simulink model "BuckDriven_DC_Mot_Offline"  (R2024b)
settings: Solver=VariableStepAuto  StartTime=0.0  StopTime=1  RelTol=1e-3
InitFcn:
  | Vin = 12;
  | 
  | %Buck Parameters
  | L = single(438e-6);
  | C = single(8e-6);
  | RDS = 0.852;
  | RL = single(0.167);
  | RD = single(0.1);
  | ESR = 2.28;
  | VD = 0.75;
  | 
  | overL = 1/L;
  | overC = 1/C;
  | 
  | %Motor Parameters
  | Ra = single(2.461);
  | La = single(0.0351);
  | Rf = single(47.74);
  | Lf = single(0.3364);
  | KLm = single(0.1963);
  | If = single(Vin/Rf);
  | J = single(0.0138);
  | f = single(0.1);
  | Tm = 0;
  | 
  | overLa = 1/La;
  | overJ = 1/J;
  | RaESR = Ra+ESR;
  | K = KLm*If;
  | 
  | vG = 4095/15;
  | wG = 4095/250;
  | 
  | h = 2e-6;
settings Model: Creator=User  LastModifiedBy=User

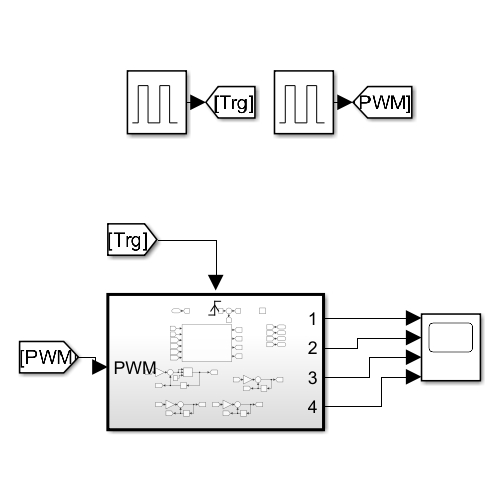
[thumbnail: Simulink's stored preview of the top-level diagram]
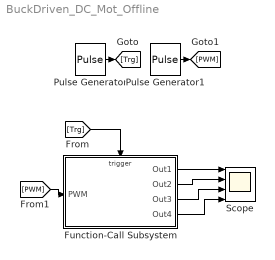
== system BuckDriven_DC_Mot_Offline ==
  Function-Call Subsystem : Subsystem  TreatAsAtomicUnit=on
  Pulse Generator : DiscretePulseGenerator  PulseType=Time based  Period=h  PulseWidth=5
  Pulse Generator1 : DiscretePulseGenerator  PulseType=Time based  Period=50e-6  PulseWidth=50
  Scope : Scope  NumInputPorts=4
  wires:
  Pulse Generator/1 -> [Trg]
  Pulse Generator1/1 -> [PWM]
  [Trg] -> Function-Call Subsystem/Trigger
  [PWM] -> Function-Call Subsystem/1(PWM)
  Function-Call Subsystem/1(Out1) -> Scope/1
  Function-Call Subsystem/2(Out2) -> Scope/2
  Function-Call Subsystem/3(Out3) -> Scope/3
  Function-Call Subsystem/4(Out4) -> Scope/4

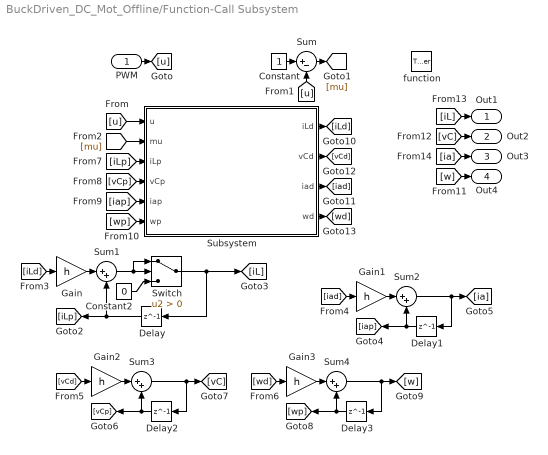
== system BuckDriven_DC_Mot_Offline/Function-Call Subsystem ==
  PWM : Inport
  function : TriggerPort  VariantControl=(inherit)
  Constant : Constant  OutDataTypeStr=single  SampleTime=-1
  Constant2 : Constant  Value=0  OutDataTypeStr=single  SampleTime=-1
  Delay{,1..3} (4 alike) : Delay  DelayLength=1
  Gain{,1..3} (4 alike) : Gain  Gain=h  OutDataTypeStr=single
  Subsystem : Subsystem
  Sum : Sum  Inputs=|+-  OutDataTypeStr=single
  Sum{1..4} (4 alike) : Sum  Inputs=|++  OutDataTypeStr=single
  Switch : Switch  Criteria=u2 > Threshold  SaturateOnIntegerOverflow=off  InputSameDT=off
  Out1 : Outport
  Out2 : Outport  Port=2
  Out3 : Outport  Port=3
  Out4 : Outport  Port=4
  wires:
  PWM/1 -> [u]
  Constant/1 -> Sum/1
  [u] -> Sum/2
  Sum/1 -> [mu]
  Gain/1 -> Sum1/1
  Delay/1 -> [iLp], Sum1/2
  [iLd] -> Gain/1
  [iad] -> Gain1/1
  Sum2/1 -> Delay1/1, [ia]
  Delay1/1 -> Sum2/2, [iap]
  Gain1/1 -> Sum2/1
  Gain2/1 -> Sum3/1
  Delay2/1 -> [vCp], Sum3/2
  Sum3/1 -> [vC], Delay2/1
  [vCd] -> Gain2/1
  [wd] -> Gain3/1
  Sum4/1 -> Delay3/1, [w]
  Delay3/1 -> Sum4/2, [wp]
  Gain3/1 -> Sum4/1
  [u] -> Subsystem/1(u)
  [mu] -> Subsystem/2(mu)
  [iLp] -> Subsystem/3(iLp)
  [vCp] -> Subsystem/4(vCp)
  [iap] -> Subsystem/5(iap)
  [wp] -> Subsystem/6(wp)
  Subsystem/1(iLd) -> [iLd]
  Subsystem/3(iad) -> [iad]
  Subsystem/2(vCd) -> [vCd]
  Subsystem/4(wd) -> [wd]
  [iL] -> Out1/1
  [vC] -> Out2/1
  [ia] -> Out3/1
  [w] -> Out4/1
  Sum1/1 -> Switch/1, Switch/2
  Constant2/1 -> Switch/3
  Switch/1 -> Delay/1, [iL]

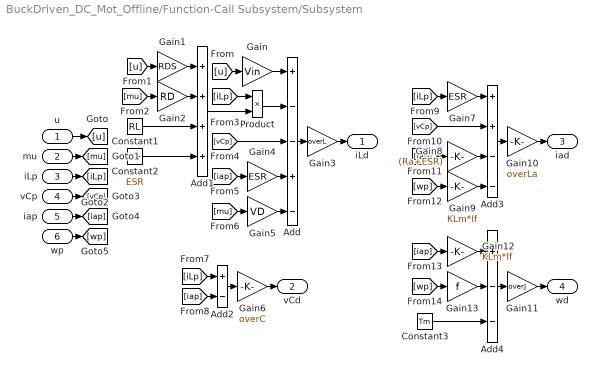
== system BuckDriven_DC_Mot_Offline/Function-Call Subsystem/Subsystem ==
  u : Inport
  mu : Inport  Port=2
  iLp : Inport  Port=3
  vCp : Inport  Port=4
  iap : Inport  Port=5
  wp : Inport  Port=6
  Add : Sum  Inputs=+--+-  OutDataTypeStr=single
  Add1 : Sum  Inputs=++++
  Add2 : Sum  Inputs=+-
  Add3 : Sum  Inputs=++--
  Add4 : Sum  Inputs=+--
  Constant1 : Constant  Value=RL  OutDataTypeStr=single  SampleTime=-1
  Constant2 : Constant  Value=ESR  OutDataTypeStr=single  SampleTime=-1
  Constant3 : Constant  Value=Tm  OutDataTypeStr=single  SampleTime=-1
  Gain : Gain  Gain=Vin  OutDataTypeStr=single
  Gain1 : Gain  Gain=RDS
  Gain10 : Gain  Gain=overLa  OutDataTypeStr=single
  Gain11 : Gain  Gain=overJ  OutDataTypeStr=single
  Gain12 : Gain  Gain=KLm*If  OutDataTypeStr=single
  Gain13 : Gain  Gain=f  OutDataTypeStr=single
  Gain2 : Gain  Gain=RD
  Gain3 : Gain  Gain=overL  OutDataTypeStr=single
  Gain4 : Gain  Gain=ESR  OutDataTypeStr=single
  Gain5 : Gain  Gain=VD  OutDataTypeStr=single
  Gain6 : Gain  Gain=overC  OutDataTypeStr=single
  Gain7 : Gain  Gain=ESR  OutDataTypeStr=single
  Gain8 : Gain  Gain=(Ra+ESR)  OutDataTypeStr=single
  Gain9 : Gain  Gain=KLm*If  OutDataTypeStr=single
  Product : Product  OutDataTypeStr=single
  iLd : Outport
  vCd : Outport  Port=2
  iad : Outport  Port=3
  wd : Outport  Port=4
  wires:
  mu/1 -> [mu]
  u/1 -> [u]
  iLp/1 -> [iLp]
  vCp/1 -> [vCp]
  iap/1 -> [iap]
  wp/1 -> [wp]
  [u] -> Gain/1
  Gain/1 -> Add/1
  Add/1 -> Gain3/1
  Gain1/1 -> Add1/1
  [u] -> Gain1/1
  Gain2/1 -> Add1/2
  [mu] -> Gain2/1
  Constant1/1 -> Add1/3
  Constant2/1 -> Add1/4
  Add1/1 -> Product/2
  [iLp] -> Product/1
  [vCp] -> Add/3
  Product/1 -> Add/2
  Gain3/1 -> iLd/1
  [iap] -> Gain4/1
  Gain4/1 -> Add/4
  [mu] -> Gain5/1
  Gain5/1 -> Add/5
  [iLp] -> Add2/1
  [iap] -> Add2/2
  Add2/1 -> Gain6/1
  Gain6/1 -> vCd/1
  Gain7/1 -> Add3/1
  [iLp] -> Gain7/1
  [vCp] -> Add3/2
  [iap] -> Gain8/1
  Gain8/1 -> Add3/3
  [wp] -> Gain9/1
  Gain9/1 -> Add3/4
  Add3/1 -> Gain10/1
  Gain10/1 -> iad/1
  Add4/1 -> Gain11/1
  Gain11/1 -> wd/1
  Gain12/1 -> Add4/1
  [iap] -> Gain12/1
  [wp] -> Gain13/1
  Gain13/1 -> Add4/2
  Constant3/1 -> Add4/3
